simulink model "salpChain36"  (Simulink 7.8)
settings: Solver=ode15s  StartTime=0.0  StopTime=400  RelTol=1e-3
values from neighbouring files (symbols this model uses):
  angleConstraintB = 25    [15RunsSmallEtta.mat]    (also in 1To10withTorque.mat; 1To20Nodes.mat; 1To30HeadToTail.mat; 1To35FullFlip.mat)
  angleConstraintK = 400    [15RunsSmallEtta.mat]    (also in 1To10withTorque.mat; 1To20Nodes.mat; 1To30HeadToTail.mat; 1To35FullFlip.mat)
  angleLimit = 90    [15RunsSmallEtta.mat]    (also in 1To10withTorque.mat; 1To20Nodes.mat; 1To30HeadToTail.mat; 1To35FullFlip.mat)
  evenTorque = [0 0 0]    [15RunsSmallEtta.mat]    (also in 1To10withTorque.mat = [0 0 0.2]; 1To20Nodes.mat; 1To30HeadToTail.mat; 1To35FullFlip.mat)
  N = size(INPUT,1)    [SpinCalc.m]
  oddTorque = [0 0 0]    [15RunsSmallEtta.mat]    (also in 1To10withTorque.mat = [0 0 0.2]; 1To20Nodes.mat; 1To30HeadToTail.mat; 1To35FullFlip.mat)
  relRotInit = [0 0]    [15RunsSmallEtta.mat]    (also in 1To10withTorque.mat; 1To20Nodes.mat; 1To30HeadToTail.mat; 1To35FullFlip.mat)
  sInertia = [0.0008  0  0; 0  0.0008  0; 0  0  0.0004]    [15RunsSmallEtta.mat]    (also in 1To10withTorque.mat; 1To20Nodes.mat; 1To30HeadToTail.mat; 1To35FullFlip.mat)
  sMass = 0.04    [15RunsSmallEtta.mat]    (also in 1To10withTorque.mat; 1To20Nodes.mat; 1To30HeadToTail.mat; 1To35FullFlip.mat)
  uAmplitudeEven = [-1.03766578533 1.19688881264 1.2209450799]    [15RunsSmallEtta.mat]    (also in 1To10withTorque.mat = [-0.2 0 2]; 1To20Nodes.mat = [-0.2 0 2]; 1To30HeadToTail.mat = [-0.2 0 2]; 1To35FullFlip.mat = [-0.2 0.2 2])
libraries: mblibv1 x613
(part 11 of 11)

== system salpChain36/Salp Odd11/2DOFJointConstrainer/AnglleConstrainer1 ==
  In1 : Inport
  Dead Zone : DeadZone  LowerValue=-angleLimit  UpperValue=angleLimit  LinearizeAsGain=off  SaturateOnIntegerOverflow=on
  Derivative : Derivative
  P : Gain  Gain=-angleConstraintK
  P1 : Gain  Gain=-angleConstraintB
  Sum : Sum  Inputs=|++
  Out1 : Outport
  wires:
  Derivative/1 -> P1/1
  P1/1 -> Sum/2
  P/1 -> Sum/1
  Sum/1 -> Out1/1
  In1/1 -> Dead Zone/1
  Dead Zone/1 -> P/1, Derivative/1

== system salpChain36/Salp Odd11/2DOFJointConstrainer/AnglleConstrainer2 ==
  In1 : Inport
  Dead Zone : DeadZone  LowerValue=-angleLimit  UpperValue=angleLimit  LinearizeAsGain=off  SaturateOnIntegerOverflow=on
  Derivative : Derivative
  P : Gain  Gain=-angleConstraintK
  P1 : Gain  Gain=-angleConstraintB
  Sum : Sum  Inputs=|++
  Out1 : Outport
  wires:
  Derivative/1 -> P1/1
  P1/1 -> Sum/2
  P/1 -> Sum/1
  Sum/1 -> Out1/1
  In1/1 -> Dead Zone/1
  Dead Zone/1 -> P/1, Derivative/1

== system salpChain36/Salp Odd12/2DOFJointConstrainer/AnglleConstrainer1 ==
  In1 : Inport
  Dead Zone : DeadZone  LowerValue=-angleLimit  UpperValue=angleLimit  LinearizeAsGain=off  SaturateOnIntegerOverflow=on
  Derivative : Derivative
  P : Gain  Gain=-angleConstraintK
  P1 : Gain  Gain=-angleConstraintB
  Sum : Sum  Inputs=|++
  Out1 : Outport
  wires:
  Derivative/1 -> P1/1
  P1/1 -> Sum/2
  P/1 -> Sum/1
  Sum/1 -> Out1/1
  In1/1 -> Dead Zone/1
  Dead Zone/1 -> P/1, Derivative/1

== system salpChain36/Salp Odd12/2DOFJointConstrainer/AnglleConstrainer2 ==
  In1 : Inport
  Dead Zone : DeadZone  LowerValue=-angleLimit  UpperValue=angleLimit  LinearizeAsGain=off  SaturateOnIntegerOverflow=on
  Derivative : Derivative
  P : Gain  Gain=-angleConstraintK
  P1 : Gain  Gain=-angleConstraintB
  Sum : Sum  Inputs=|++
  Out1 : Outport
  wires:
  Derivative/1 -> P1/1
  P1/1 -> Sum/2
  P/1 -> Sum/1
  Sum/1 -> Out1/1
  In1/1 -> Dead Zone/1
  Dead Zone/1 -> P/1, Derivative/1

== system salpChain36/Salp Odd2/2DOFJointConstrainer/AnglleConstrainer1 ==
  In1 : Inport
  Dead Zone : DeadZone  LowerValue=-angleLimit  UpperValue=angleLimit  LinearizeAsGain=off  SaturateOnIntegerOverflow=on
  Derivative : Derivative
  P : Gain  Gain=-angleConstraintK
  P1 : Gain  Gain=-angleConstraintB
  Sum : Sum  Inputs=|++
  Out1 : Outport
  wires:
  Derivative/1 -> P1/1
  P1/1 -> Sum/2
  P/1 -> Sum/1
  Sum/1 -> Out1/1
  In1/1 -> Dead Zone/1
  Dead Zone/1 -> P/1, Derivative/1

== system salpChain36/Salp Odd2/2DOFJointConstrainer/AnglleConstrainer2 ==
  In1 : Inport
  Dead Zone : DeadZone  LowerValue=-angleLimit  UpperValue=angleLimit  LinearizeAsGain=off  SaturateOnIntegerOverflow=on
  Derivative : Derivative
  P : Gain  Gain=-angleConstraintK
  P1 : Gain  Gain=-angleConstraintB
  Sum : Sum  Inputs=|++
  Out1 : Outport
  wires:
  Derivative/1 -> P1/1
  P1/1 -> Sum/2
  P/1 -> Sum/1
  Sum/1 -> Out1/1
  In1/1 -> Dead Zone/1
  Dead Zone/1 -> P/1, Derivative/1

== system salpChain36/Salp Odd3/2DOFJointConstrainer/AnglleConstrainer1 ==
  In1 : Inport
  Dead Zone : DeadZone  LowerValue=-angleLimit  UpperValue=angleLimit  LinearizeAsGain=off  SaturateOnIntegerOverflow=on
  Derivative : Derivative
  P : Gain  Gain=-angleConstraintK
  P1 : Gain  Gain=-angleConstraintB
  Sum : Sum  Inputs=|++
  Out1 : Outport
  wires:
  Derivative/1 -> P1/1
  P1/1 -> Sum/2
  P/1 -> Sum/1
  Sum/1 -> Out1/1
  In1/1 -> Dead Zone/1
  Dead Zone/1 -> P/1, Derivative/1

== system salpChain36/Salp Odd3/2DOFJointConstrainer/AnglleConstrainer2 ==
  In1 : Inport
  Dead Zone : DeadZone  LowerValue=-angleLimit  UpperValue=angleLimit  LinearizeAsGain=off  SaturateOnIntegerOverflow=on
  Derivative : Derivative
  P : Gain  Gain=-angleConstraintK
  P1 : Gain  Gain=-angleConstraintB
  Sum : Sum  Inputs=|++
  Out1 : Outport
  wires:
  Derivative/1 -> P1/1
  P1/1 -> Sum/2
  P/1 -> Sum/1
  Sum/1 -> Out1/1
  In1/1 -> Dead Zone/1
  Dead Zone/1 -> P/1, Derivative/1

== system salpChain36/Salp Odd4/2DOFJointConstrainer/AnglleConstrainer1 ==
  In1 : Inport
  Dead Zone : DeadZone  LowerValue=-angleLimit  UpperValue=angleLimit  LinearizeAsGain=off  SaturateOnIntegerOverflow=on
  Derivative : Derivative
  P : Gain  Gain=-angleConstraintK
  P1 : Gain  Gain=-angleConstraintB
  Sum : Sum  Inputs=|++
  Out1 : Outport
  wires:
  Derivative/1 -> P1/1
  P1/1 -> Sum/2
  P/1 -> Sum/1
  Sum/1 -> Out1/1
  In1/1 -> Dead Zone/1
  Dead Zone/1 -> P/1, Derivative/1

== system salpChain36/Salp Odd4/2DOFJointConstrainer/AnglleConstrainer2 ==
  In1 : Inport
  Dead Zone : DeadZone  LowerValue=-angleLimit  UpperValue=angleLimit  LinearizeAsGain=off  SaturateOnIntegerOverflow=on
  Derivative : Derivative
  P : Gain  Gain=-angleConstraintK
  P1 : Gain  Gain=-angleConstraintB
  Sum : Sum  Inputs=|++
  Out1 : Outport
  wires:
  Derivative/1 -> P1/1
  P1/1 -> Sum/2
  P/1 -> Sum/1
  Sum/1 -> Out1/1
  In1/1 -> Dead Zone/1
  Dead Zone/1 -> P/1, Derivative/1

== system salpChain36/Salp Odd5/2DOFJointConstrainer/AnglleConstrainer1 ==
  In1 : Inport
  Dead Zone : DeadZone  LowerValue=-angleLimit  UpperValue=angleLimit  LinearizeAsGain=off  SaturateOnIntegerOverflow=on
  Derivative : Derivative
  P : Gain  Gain=-angleConstraintK
  P1 : Gain  Gain=-angleConstraintB
  Sum : Sum  Inputs=|++
  Out1 : Outport
  wires:
  Derivative/1 -> P1/1
  P1/1 -> Sum/2
  P/1 -> Sum/1
  Sum/1 -> Out1/1
  In1/1 -> Dead Zone/1
  Dead Zone/1 -> P/1, Derivative/1

== system salpChain36/Salp Odd5/2DOFJointConstrainer/AnglleConstrainer2 ==
  In1 : Inport
  Dead Zone : DeadZone  LowerValue=-angleLimit  UpperValue=angleLimit  LinearizeAsGain=off  SaturateOnIntegerOverflow=on
  Derivative : Derivative
  P : Gain  Gain=-angleConstraintK
  P1 : Gain  Gain=-angleConstraintB
  Sum : Sum  Inputs=|++
  Out1 : Outport
  wires:
  Derivative/1 -> P1/1
  P1/1 -> Sum/2
  P/1 -> Sum/1
  Sum/1 -> Out1/1
  In1/1 -> Dead Zone/1
  Dead Zone/1 -> P/1, Derivative/1

== system salpChain36/Salp Odd6/2DOFJointConstrainer/AnglleConstrainer1 ==
  In1 : Inport
  Dead Zone : DeadZone  LowerValue=-angleLimit  UpperValue=angleLimit  LinearizeAsGain=off  SaturateOnIntegerOverflow=on
  Derivative : Derivative
  P : Gain  Gain=-angleConstraintK
  P1 : Gain  Gain=-angleConstraintB
  Sum : Sum  Inputs=|++
  Out1 : Outport
  wires:
  Derivative/1 -> P1/1
  P1/1 -> Sum/2
  P/1 -> Sum/1
  Sum/1 -> Out1/1
  In1/1 -> Dead Zone/1
  Dead Zone/1 -> P/1, Derivative/1

== system salpChain36/Salp Odd6/2DOFJointConstrainer/AnglleConstrainer2 ==
  In1 : Inport
  Dead Zone : DeadZone  LowerValue=-angleLimit  UpperValue=angleLimit  LinearizeAsGain=off  SaturateOnIntegerOverflow=on
  Derivative : Derivative
  P : Gain  Gain=-angleConstraintK
  P1 : Gain  Gain=-angleConstraintB
  Sum : Sum  Inputs=|++
  Out1 : Outport
  wires:
  Derivative/1 -> P1/1
  P1/1 -> Sum/2
  P/1 -> Sum/1
  Sum/1 -> Out1/1
  In1/1 -> Dead Zone/1
  Dead Zone/1 -> P/1, Derivative/1

== system salpChain36/Salp Odd7/2DOFJointConstrainer/AnglleConstrainer1 ==
  In1 : Inport
  Dead Zone : DeadZone  LowerValue=-angleLimit  UpperValue=angleLimit  LinearizeAsGain=off  SaturateOnIntegerOverflow=on
  Derivative : Derivative
  P : Gain  Gain=-angleConstraintK
  P1 : Gain  Gain=-angleConstraintB
  Sum : Sum  Inputs=|++
  Out1 : Outport
  wires:
  Derivative/1 -> P1/1
  P1/1 -> Sum/2
  P/1 -> Sum/1
  Sum/1 -> Out1/1
  In1/1 -> Dead Zone/1
  Dead Zone/1 -> P/1, Derivative/1

== system salpChain36/Salp Odd7/2DOFJointConstrainer/AnglleConstrainer2 ==
  In1 : Inport
  Dead Zone : DeadZone  LowerValue=-angleLimit  UpperValue=angleLimit  LinearizeAsGain=off  SaturateOnIntegerOverflow=on
  Derivative : Derivative
  P : Gain  Gain=-angleConstraintK
  P1 : Gain  Gain=-angleConstraintB
  Sum : Sum  Inputs=|++
  Out1 : Outport
  wires:
  Derivative/1 -> P1/1
  P1/1 -> Sum/2
  P/1 -> Sum/1
  Sum/1 -> Out1/1
  In1/1 -> Dead Zone/1
  Dead Zone/1 -> P/1, Derivative/1

== system salpChain36/Salp Odd8/2DOFJointConstrainer/AnglleConstrainer1 ==
  In1 : Inport
  Dead Zone : DeadZone  LowerValue=-angleLimit  UpperValue=angleLimit  LinearizeAsGain=off  SaturateOnIntegerOverflow=on
  Derivative : Derivative
  P : Gain  Gain=-angleConstraintK
  P1 : Gain  Gain=-angleConstraintB
  Sum : Sum  Inputs=|++
  Out1 : Outport
  wires:
  Derivative/1 -> P1/1
  P1/1 -> Sum/2
  P/1 -> Sum/1
  Sum/1 -> Out1/1
  In1/1 -> Dead Zone/1
  Dead Zone/1 -> P/1, Derivative/1

== system salpChain36/Salp Odd8/2DOFJointConstrainer/AnglleConstrainer2 ==
  In1 : Inport
  Dead Zone : DeadZone  LowerValue=-angleLimit  UpperValue=angleLimit  LinearizeAsGain=off  SaturateOnIntegerOverflow=on
  Derivative : Derivative
  P : Gain  Gain=-angleConstraintK
  P1 : Gain  Gain=-angleConstraintB
  Sum : Sum  Inputs=|++
  Out1 : Outport
  wires:
  Derivative/1 -> P1/1
  P1/1 -> Sum/2
  P/1 -> Sum/1
  Sum/1 -> Out1/1
  In1/1 -> Dead Zone/1
  Dead Zone/1 -> P/1, Derivative/1

== system salpChain36/Salp Odd9/2DOFJointConstrainer/AnglleConstrainer1 ==
  In1 : Inport
  Dead Zone : DeadZone  LowerValue=-angleLimit  UpperValue=angleLimit  LinearizeAsGain=off  SaturateOnIntegerOverflow=on
  Derivative : Derivative
  P : Gain  Gain=-angleConstraintK
  P1 : Gain  Gain=-angleConstraintB
  Sum : Sum  Inputs=|++
  Out1 : Outport
  wires:
  Derivative/1 -> P1/1
  P1/1 -> Sum/2
  P/1 -> Sum/1
  Sum/1 -> Out1/1
  In1/1 -> Dead Zone/1
  Dead Zone/1 -> P/1, Derivative/1

== system salpChain36/Salp Odd9/2DOFJointConstrainer/AnglleConstrainer2 ==
  In1 : Inport
  Dead Zone : DeadZone  LowerValue=-angleLimit  UpperValue=angleLimit  LinearizeAsGain=off  SaturateOnIntegerOverflow=on
  Derivative : Derivative
  P : Gain  Gain=-angleConstraintK
  P1 : Gain  Gain=-angleConstraintB
  Sum : Sum  Inputs=|++
  Out1 : Outport
  wires:
  Derivative/1 -> P1/1
  P1/1 -> Sum/2
  P/1 -> Sum/1
  Sum/1 -> Out1/1
  In1/1 -> Dead Zone/1
  Dead Zone/1 -> P/1, Derivative/1

== system salpChain36/preEnd Salp Odd/2DOFJointConstrainer/AnglleConstrainer1 ==
  In1 : Inport
  Dead Zone : DeadZone  LowerValue=-angleLimit  UpperValue=angleLimit  LinearizeAsGain=off  SaturateOnIntegerOverflow=on
  Derivative : Derivative
  P : Gain  Gain=-angleConstraintK
  P1 : Gain  Gain=-angleConstraintB
  Sum : Sum  Inputs=|++
  Out1 : Outport
  wires:
  Derivative/1 -> P1/1
  P1/1 -> Sum/2
  P/1 -> Sum/1
  Sum/1 -> Out1/1
  In1/1 -> Dead Zone/1
  Dead Zone/1 -> P/1, Derivative/1

== system salpChain36/preEnd Salp Odd/2DOFJointConstrainer/AnglleConstrainer2 ==
  In1 : Inport
  Dead Zone : DeadZone  LowerValue=-angleLimit  UpperValue=angleLimit  LinearizeAsGain=off  SaturateOnIntegerOverflow=on
  Derivative : Derivative
  P : Gain  Gain=-angleConstraintK
  P1 : Gain  Gain=-angleConstraintB
  Sum : Sum  Inputs=|++
  Out1 : Outport
  wires:
  Derivative/1 -> P1/1
  P1/1 -> Sum/2
  P/1 -> Sum/1
  Sum/1 -> Out1/1
  In1/1 -> Dead Zone/1
  Dead Zone/1 -> P/1, Derivative/1
